simulink model "twolinkarm"  (R2017a)
settings: Solver=VariableStepAuto  StartTime=0.0  StopTime=tTotal  FixedStep=1e-6  MinStep=1e-8  RelTol=1e-3
values from neighbouring files (symbols this model uses):
  a1_val = 0.05    [twolinkarm_init.m]
  a2_val = 0.05    [twolinkarm_init.m]
  Jm = 3.2284E-6    (= 3.2284e-06)    [twolinkarm_init.m]
  lC1_val = a1_val/2    (= 0.025)    [twolinkarm_init.m]
  lC2_val = a2_val/2    (= 0.025)    [twolinkarm_init.m]
  mL1_val = 0.01    [twolinkarm_init.m]
  mL2_val = 0.01    [twolinkarm_init.m]
  ts = 0.1    [twolinkarm_init.m]
  V = 7.4    [twolinkarm_init.m]
  Y = simplify(Y)    [twolinkarm_DPI1.m]    (also in twolinkarm_DPI2.m = subs(Y, [lC1, lC2],[0.5*a1, 0.5*a2]); twolinkarm_init.m = subs(Y,      [a1, a2, lC1, lC2, k1, k2],      [a1_val, a2_va)
undefined symbols (not defined in the file or in its folder): Ry, X, Z
libraries: sm_lib x13, nesl_utility x11, fl_lib x10, elec_lib x2
settings Model: Creator=ashlin  LastModifiedBy=ashlin
settings SolverCC: ZeroCrossAlgorithm=Adaptive
settings DataIOCC: SaveFormat=Array
settings DiagnosticsConfigSet: SimMechanicsUnconnectedFramePorts=none  SimMechanicsUnconnectedGeometryPorts=none

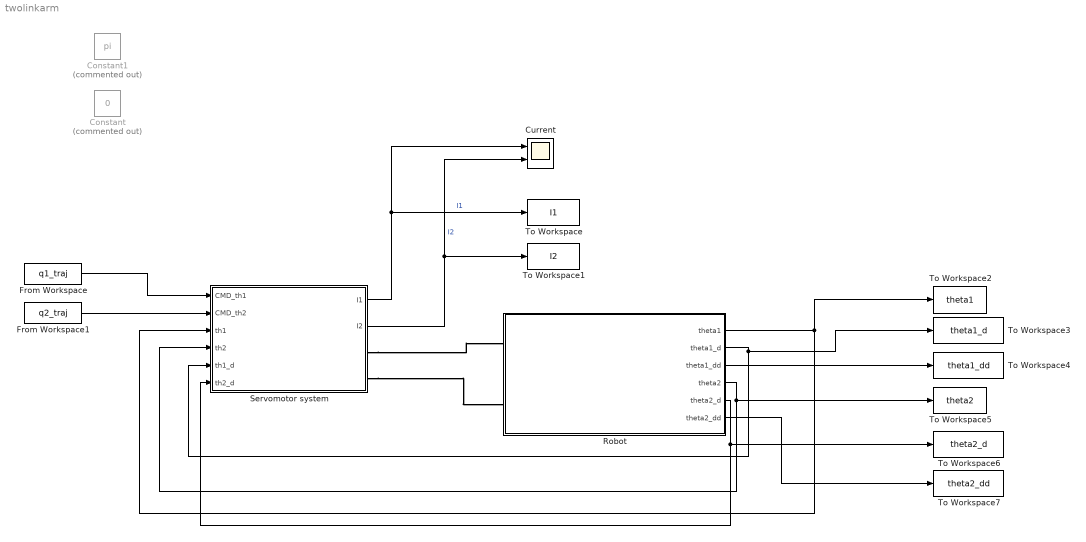
== system twolinkarm ==
  Constant : Constant  Commented=on  Value=0
  Constant1 : Constant  Commented=on  Value=pi
  Current : Scope  NumInputPorts=2
  From Workspace : FromWorkspace  VariableName=q1_traj  SampleTime=0
  From Workspace1 : FromWorkspace  VariableName=q2_traj  SampleTime=0
  Robot : Subsystem
  Servomotor system : Subsystem
  To Workspace : ToWorkspace  VariableName=I1  SaveFormat=Timeseries  SampleTime=ts
  To Workspace1 : ToWorkspace  VariableName=I2  SaveFormat=Timeseries  SampleTime=ts
  To Workspace2 : ToWorkspace  VariableName=theta1  SaveFormat=Timeseries  SampleTime=ts
  To Workspace3 : ToWorkspace  VariableName=theta1_d  SaveFormat=Timeseries  SampleTime=ts
  To Workspace4 : ToWorkspace  VariableName=theta1_dd  SaveFormat=Timeseries  SampleTime=ts
  To Workspace5 : ToWorkspace  VariableName=theta2  SaveFormat=Timeseries  SampleTime=ts
  To Workspace6 : ToWorkspace  VariableName=theta2_d  SaveFormat=Timeseries  SampleTime=ts
  To Workspace7 : ToWorkspace  VariableName=theta2_dd  SaveFormat=Timeseries  SampleTime=ts
  wires:
  Servomotor system/1(I1) -> To Workspace/1, Current/1  "I1"
  Servomotor system/2(I2) -> To Workspace1/1, Current/2  "I2"
  Robot/1(theta1) -> To Workspace2/1, Servomotor system/3(th1)
  Robot/2(theta1_d) -> To Workspace3/1, Servomotor system/5(th1_d)
  Robot/3(theta1_dd) -> To Workspace4/1
  Robot/5(theta2_d) -> To Workspace6/1, Servomotor system/6(th2_d)
  Robot/6(theta2_dd) -> To Workspace7/1
  Robot/4(theta2) -> Servomotor system/4(th2), To Workspace5/1
  From Workspace/1 -> Servomotor system/1(CMD_th1)
  From Workspace1/1 -> Servomotor system/2(CMD_th2)
  connections:
  Servomotor system/RConn1 -- Robot/LConn1
  Servomotor system/RConn2 -- Robot/LConn2

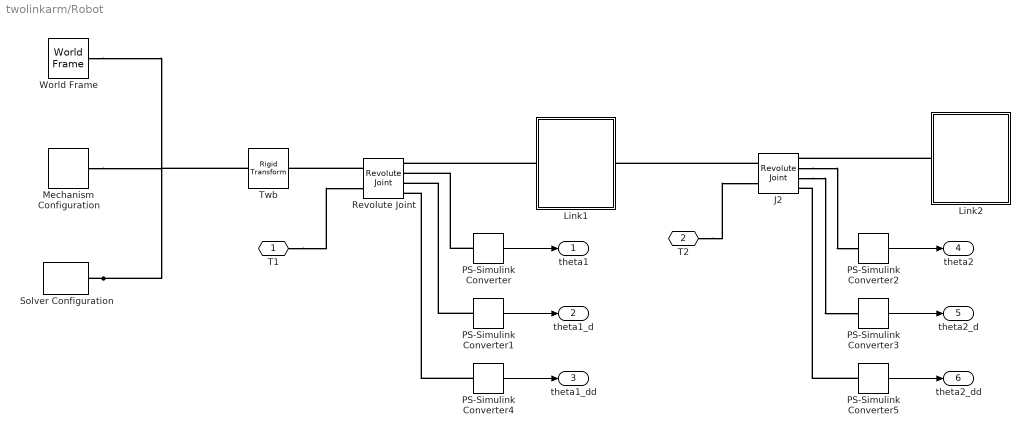
== system twolinkarm/Robot ==
  J2 : sm_lib/Joints/Revolute Joint  SenseConstraintForce=off  SenseConstraintForceX=off  SenseConstraintForceY=off  SenseConstraintForceZ=off  SenseConstraintTorque=off  SenseConstraintTorqueX=off  SenseConstraintTorqueY=off  SenseConstraintTorqueZ=off  SenseTotalForce=off  SenseTotalForceX=off  SenseTotalForceY=off  SenseTotalForceZ=off  SenseTotalTorque=off  SenseTotalTorqueX=off  SenseTotalTorqueY=off  SenseTotalTorqueZ=off  CompositeWrenchDir=FollowerOnBase  CompositeWrenchFrame=BaseFrame  EquilibriumPosition=0  EquilibriumPositionUnits=deg  SpringStiffness=0  SpringStiffnessUnits=N*m/deg  DampingCoefficient=0  DampingCoefficientUnits=N*m/(deg/s)  TorqueActuationMode=InputTorque  MotionActuationMode=ComputedMotion  SensePosition=on  SenseVelocity=on  SenseAcceleration=on  SenseTorqueForce=off  PositionTargetSpecify=off  PositionTargetPriority=High  PositionTargetValue=0  PositionTargetValueUnits=deg  VelocityTargetSpecify=off  VelocityTargetPriority=High  VelocityTargetValue=0  VelocityTargetValueUnits=deg/s
  Link1 : Subsystem
  Link2 : Subsystem
  Mechanism Configuration : sm_lib/Utilities/Mechanism Configuration  UniformGravity=Constant  GravityVector=[0 -9.81 0]  GravityUnits=m/s^2  LinearizationDelta=0.001
  PS-Simulink Converter{,1..5} (6 alike) : nesl_utility/PS-Simulink Converter  PhysicalDomain=network_engine_domain  SubClassName=ps_output  LeftPortType=input  RightPortType=output  PseudoPeriodic=off  Frequencies=[]  Unit=1  AffineConversion=off
  Revolute Joint : sm_lib/Joints/Revolute Joint  SenseConstraintForce=off  SenseConstraintForceX=off  SenseConstraintForceY=off  SenseConstraintForceZ=off  SenseConstraintTorque=off  SenseConstraintTorqueX=off  SenseConstraintTorqueY=off  SenseConstraintTorqueZ=off  SenseTotalForce=off  SenseTotalForceX=off  SenseTotalForceY=off  SenseTotalForceZ=off  SenseTotalTorque=off  SenseTotalTorqueX=off  SenseTotalTorqueY=off  SenseTotalTorqueZ=off  CompositeWrenchDir=FollowerOnBase  CompositeWrenchFrame=BaseFrame  EquilibriumPosition=0  EquilibriumPositionUnits=deg  SpringStiffness=0  SpringStiffnessUnits=N*m/deg  DampingCoefficient=0  DampingCoefficientUnits=N*m/(deg/s)  TorqueActuationMode=InputTorque  MotionActuationMode=ComputedMotion  SensePosition=on  SenseVelocity=on  SenseAcceleration=on  SenseTorqueForce=off  PositionTargetSpecify=off  PositionTargetPriority=High  PositionTargetValue=0  PositionTargetValueUnits=deg  VelocityTargetSpecify=off  VelocityTargetPriority=High  VelocityTargetValue=0  VelocityTargetValueUnits=deg/s
  Solver Configuration : nesl_utility/Solver Configuration  PhysicalDomain=network_engine_domain  SubClassName=solver  LeftPortType=input  RightPortType=generic  Accelerate=off  Tones=[]  Harmonics=[]  SimulateNoise=off  Profile=off  UseLocalSampling=off  EnableSwitchedLinearOptims=on  FrequencyDomain=off  UseCCode=off  RelTol=0.001  AbsTol=1e-06  MinStep=1e-09  ToWorkspace=off  RevertToSquareIcSolve=off  NumHomotopyIterations=100  PhasorMode=off  PhasorModeNumHarmonics=1  OverrideAbsTol=off  DoDC=off  ResidualTolerance=1e-04  UseLocalSolver=off  LocalSolverChoice=NE_BACKWARD_EULER_ADVANCER  LocalSolverSampleTime=0.001  DoFixedCost=off  MaxNonlinIter=3  MaxModeIter=2  LinearAlgebra=Sparse  DelaysMemoryBudget=1024  AutomaticFiltering=on  FilteringTimeConstant=0.001
  Twb : sm_lib/Frames and Transforms/Rigid Transform  TranslationMethod=None  TranslationStandardOffset=0  TranslationLengthUnit=m  TranslationStandardAxis=+Z  TranslationCartesianOffset=[0 0 0]  TranslationROffset=0  TranslationROffsetUnits=m  TranslationZOffset=0  TranslationZOffsetUnits=m  TranslationThetaOffset=0  TranslationThetaOffsetUnits=deg  RotationMethod=None  RotationAngleUnits=deg  RotationStandardAxis=+Z  RotationAngle=0.0  RotationArbitraryAxis=[0 0 1]  FollAlignAxisA=+X  BaseAlignAxisA=+Y  FollAlignAxisB=+Y  BaseAlignAxisB=+Z  RotationSequenceAxes=FollowerAxes  RotationSequence=XYX  RotationSequenceAngles=[0 0 0]  RotationSequenceAnglesUnits=deg  RotationMatrix=eye(3,3)
  World Frame : sm_lib/Frames and Transforms/World Frame
  T1 : PMIOPort  Port=1  Side=Left
  T2 : PMIOPort  Port=2  Side=Left
  theta1 : Outport
  theta1_d : Outport  Port=2
  theta1_dd : Outport  Port=3
  theta2 : Outport  Port=4
  theta2_d : Outport  Port=5
  theta2_dd : Outport  Port=6
  wires:
  PS-Simulink Converter/1 -> theta1/1
  PS-Simulink Converter1/1 -> theta1_d/1
  PS-Simulink Converter3/1 -> theta2_d/1
  PS-Simulink Converter2/1 -> theta2/1
  PS-Simulink Converter4/1 -> theta1_dd/1
  PS-Simulink Converter5/1 -> theta2_dd/1
  connections:
  Solver Configuration/RConn1 -- World Frame/RConn1 -- Twb/LConn1 -- Mechanism Configuration/RConn1
  PS-Simulink Converter/LConn1 -- Revolute Joint/RConn2
  T1/RConn1 -- Revolute Joint/LConn2
  Link1/LConn1 -- Revolute Joint/RConn1
  Revolute Joint/LConn1 -- Twb/RConn1
  J2/LConn1 -- Link1/RConn1
  T2/RConn1 -- J2/LConn2
  Link2/LConn1 -- J2/RConn1
  PS-Simulink Converter1/LConn1 -- Revolute Joint/RConn3
  J2/RConn2 -- PS-Simulink Converter2/LConn1
  J2/RConn3 -- PS-Simulink Converter3/LConn1
  PS-Simulink Converter4/LConn1 -- Revolute Joint/RConn4
  PS-Simulink Converter5/LConn1 -- J2/RConn4

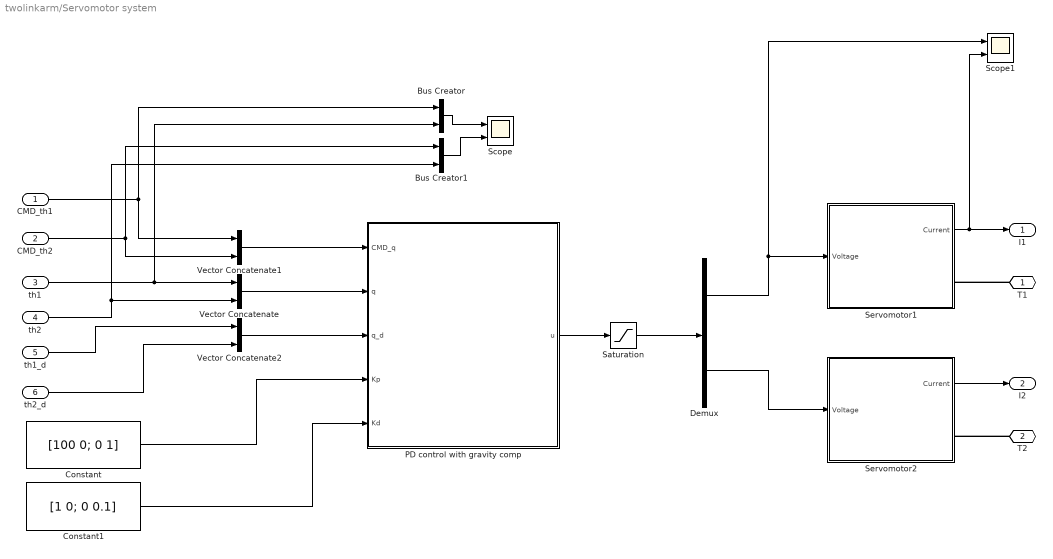
== system twolinkarm/Servomotor system ==
  CMD_th1 : Inport
  CMD_th2 : Inport  Port=2
  th1 : Inport  Port=3
  th2 : Inport  Port=4
  th1_d : Inport  Port=5
  th2_d : Inport  Port=6
  Bus Creator : BusCreator  Inputs=2
  Bus Creator1 : BusCreator  Inputs=2
  Constant : Constant  Value=[100 0; 0 1]
  Constant1 : Constant  Value=[1 0; 0 0.1]
  Demux : Demux  Outputs=2
  PD control with gravity comp : Subsystem
  Saturation : Saturate  UpperLimit=[V; V]  LowerLimit=[-V; -V]
  Scope : Scope  NumInputPorts=2
  Scope1 : Scope  NumInputPorts=2
  Servomotor1 : Subsystem
  Servomotor2 : Subsystem
  Vector Concatenate : Concatenate
  Vector Concatenate1 : Concatenate
  Vector Concatenate2 : Concatenate
  T1 : PMIOPort  Port=1  Side=Right
  T2 : PMIOPort  Port=2  Side=Right
  I1 : Outport
  I2 : Outport  Port=2
  wires:
  th1/1 -> Vector Concatenate/1, Bus Creator/2
  CMD_th1/1 -> Vector Concatenate1/1, Bus Creator/1
  Servomotor1/1(Current) -> Scope1/2, I1/1
  CMD_th2/1 -> Vector Concatenate1/2, Bus Creator1/1
  Servomotor2/1(Current) -> I2/1
  Demux/2 -> Servomotor2/1(Voltage)
  th2/1 -> Bus Creator1/2, Vector Concatenate/2
  Bus Creator1/1 -> Scope/2
  Bus Creator/1 -> Scope/1
  PD control with gravity comp/1(u) -> Saturation/1
  Vector Concatenate/1 -> PD control with gravity comp/2(q)
  Vector Concatenate1/1 -> PD control with gravity comp/1(CMD_q)
  Vector Concatenate2/1 -> PD control with gravity comp/3(q_d)
  th2_d/1 -> Vector Concatenate2/2
  th1_d/1 -> Vector Concatenate2/1
  Constant/1 -> PD control with gravity comp/4(Kp)
  Constant1/1 -> PD control with gravity comp/5(Kd)
  Demux/1 -> Scope1/1, Servomotor1/1(Voltage)
  Saturation/1 -> Demux/1
  connections:
  T1/RConn1 -- Servomotor1/RConn1
  T2/RConn1 -- Servomotor2/RConn1

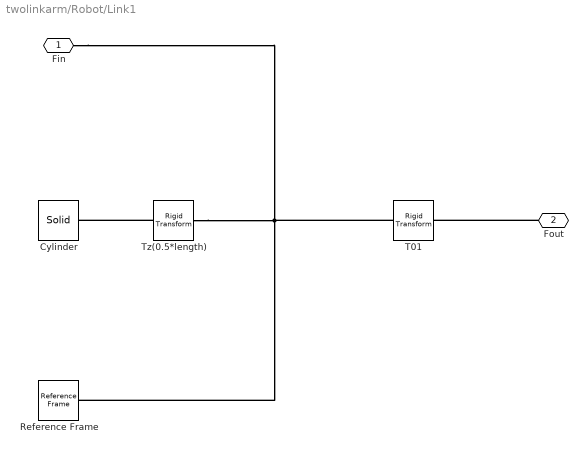
== system twolinkarm/Robot/Link1 ==
  Cylinder : sm_lib/Body Elements/Solid  InertiaType=CalculateFromGeometry  Mass=1  MassUnits=kg  CenterOfMass=[0 0 0]  CenterOfMassUnits=m  MomentsOfInertia=[1 1 1]  MomentsOfInertiaUnits=kg*m^2  ProductsOfInertia=[1 1 1]  ProductsOfInertiaUnits=kg*m^2  DensityBased=on  Density=density  DensityUnits=kg/m^3  DoExposeReferenceFrame=on  SerializedFrames=<Frames/>  GraphicType=FromGeometry  MarkerShape=Sphere  MarkerSize=10  GraphicVisPropType=SimpleVisualProperties  GraphicDiffuseColor=[0.0 1.0 0.4]  GraphicSpecularColor=[0.5 0.5 0.5 1.0]  GraphicAmbientColor=[0.15 0.15 0.15 1.0]  GraphicEmissiveColor=[0.0 0.0 0.0 1.0]  GraphicShininess=75  GraphicOpacity=1.0  GeometryShape=Cylinder  RectangleSize=[1 1]  RectangleSizeUnits=m  BrickDimensions=[1 1 1]  BrickDimensionUnits=m  CylinderRadius=rLink  CylinderRadiusUnits=m  CylinderLength=a1_val  CylinderLengthUnits=m  SphereRadius=1  SphereRadiusUnits=m  EllipsoidRadii=[1 1 1]  EllipsoidRadiiUnits=m  ExtrusionCrossSection=[1 1; -1 1; -1 -1; 1 -1]  ExtrusionCrossSectionUnits=m  ExtrusionLength=1  ExtrusionLengthUnits=m  PolygonNumSides=3  PolygonOuterRadius=1  PolygonOuterRadiusUnits=m  ExtGeomFileType=STEP  ExtGeomFileUnits=m  RevolutionCrossSection=[1 1; 1 -1; 2 -1; 2 1]  RevolutionCrossSectionUnits=m  RevolutionExtent=Full  RevolutionAngle=180  RevolutionAngleUnits=deg
  Reference Frame : sm_lib/Frames and Transforms/Reference Frame
  T01 : sm_lib/Frames and Transforms/Rigid Transform  TranslationMethod=Cartesian  TranslationStandardOffset=0.1/2  TranslationLengthUnit=m  TranslationStandardAxis=+Z  TranslationCartesianOffset=[a1_val 0 0]  TranslationROffset=0  TranslationROffsetUnits=m  TranslationZOffset=0  TranslationZOffsetUnits=m  TranslationThetaOffset=0  TranslationThetaOffsetUnits=deg  RotationMethod=RotationMatrix  RotationAngleUnits=deg  RotationStandardAxis=+Y  RotationAngle=90  RotationArbitraryAxis=[0 0 1]  FollAlignAxisA=+X  BaseAlignAxisA=+Y  FollAlignAxisB=+Y  BaseAlignAxisB=+Z  RotationSequenceAxes=FollowerAxes  RotationSequence=XYX  RotationSequenceAngles=[0 0 0]  RotationSequenceAnglesUnits=deg  RotationMatrix=eye(3,3)
  Tz(0.5*length) : sm_lib/Frames and Transforms/Rigid Transform  TranslationMethod=Cartesian  TranslationStandardOffset=0  TranslationLengthUnit=m  TranslationStandardAxis=-X  TranslationCartesianOffset=[ 0 0 -a1_val/2]  TranslationROffset=0  TranslationROffsetUnits=m  TranslationZOffset=0  TranslationZOffsetUnits=m  TranslationThetaOffset=0  TranslationThetaOffsetUnits=deg  RotationMethod=RotationMatrix  RotationAngleUnits=deg  RotationStandardAxis=+Z  RotationAngle=0.0  RotationArbitraryAxis=[0 0 1]  FollAlignAxisA=+X  BaseAlignAxisA=+Y  FollAlignAxisB=+Y  BaseAlignAxisB=+Z  RotationSequenceAxes=FollowerAxes  RotationSequence=XYX  RotationSequenceAngles=[0 0 0]  RotationSequenceAnglesUnits=deg  RotationMatrix=Ry(pi/2)
  Fin : PMIOPort  Port=1  Side=Left
  Fout : PMIOPort  Port=2  Side=Right
  connections:
  Tz(0.5*length)/LConn1 -- Cylinder/RConn1
  Fin/RConn1 -- T01/LConn1 -- Tz(0.5*length)/RConn1 -- Reference Frame/RConn1
  Fout/RConn1 -- T01/RConn1

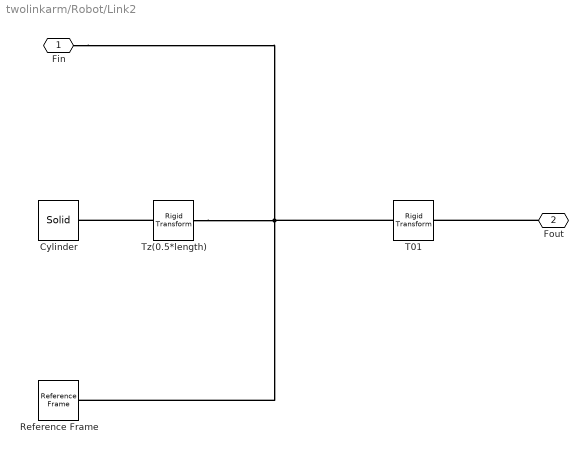
== system twolinkarm/Robot/Link2 ==
  Cylinder : sm_lib/Body Elements/Solid  InertiaType=CalculateFromGeometry  Mass=1  MassUnits=kg  CenterOfMass=[0 0 0]  CenterOfMassUnits=m  MomentsOfInertia=[1 1 1]  MomentsOfInertiaUnits=kg*m^2  ProductsOfInertia=[1 1 1]  ProductsOfInertiaUnits=kg*m^2  DensityBased=on  Density=density  DensityUnits=kg/m^3  DoExposeReferenceFrame=on  SerializedFrames=<Frames/>  GraphicType=FromGeometry  MarkerShape=Sphere  MarkerSize=10  GraphicVisPropType=SimpleVisualProperties  GraphicDiffuseColor=[0.0 1.0 0.4]  GraphicSpecularColor=[0.5 0.5 0.5 1.0]  GraphicAmbientColor=[0.15 0.15 0.15 1.0]  GraphicEmissiveColor=[0.0 0.0 0.0 1.0]  GraphicShininess=75  GraphicOpacity=1.0  GeometryShape=Cylinder  RectangleSize=[1 1]  RectangleSizeUnits=m  BrickDimensions=[1 1 1]  BrickDimensionUnits=m  CylinderRadius=rLink  CylinderRadiusUnits=m  CylinderLength=a2_val  CylinderLengthUnits=m  SphereRadius=1  SphereRadiusUnits=m  EllipsoidRadii=[1 1 1]  EllipsoidRadiiUnits=m  ExtrusionCrossSection=[1 1; -1 1; -1 -1; 1 -1]  ExtrusionCrossSectionUnits=m  ExtrusionLength=1  ExtrusionLengthUnits=m  PolygonNumSides=3  PolygonOuterRadius=1  PolygonOuterRadiusUnits=m  ExtGeomFileType=STEP  ExtGeomFileUnits=m  RevolutionCrossSection=[1 1; 1 -1; 2 -1; 2 1]  RevolutionCrossSectionUnits=m  RevolutionExtent=Full  RevolutionAngle=180  RevolutionAngleUnits=deg
  Reference Frame : sm_lib/Frames and Transforms/Reference Frame
  T01 : sm_lib/Frames and Transforms/Rigid Transform  TranslationMethod=Cartesian  TranslationStandardOffset=0.1/2  TranslationLengthUnit=m  TranslationStandardAxis=+Z  TranslationCartesianOffset=[a2_val 0 0]  TranslationROffset=0  TranslationROffsetUnits=m  TranslationZOffset=0  TranslationZOffsetUnits=m  TranslationThetaOffset=0  TranslationThetaOffsetUnits=deg  RotationMethod=RotationMatrix  RotationAngleUnits=deg  RotationStandardAxis=+Y  RotationAngle=90  RotationArbitraryAxis=[0 0 1]  FollAlignAxisA=+X  BaseAlignAxisA=+Y  FollAlignAxisB=+Y  BaseAlignAxisB=+Z  RotationSequenceAxes=FollowerAxes  RotationSequence=XYX  RotationSequenceAngles=[0 0 0]  RotationSequenceAnglesUnits=deg  RotationMatrix=eye(3,3)
  Tz(0.5*length) : sm_lib/Frames and Transforms/Rigid Transform  TranslationMethod=StandardAxis  TranslationStandardOffset=a2_val/2  TranslationLengthUnit=m  TranslationStandardAxis=-Z  TranslationCartesianOffset=[ 0 0 -0.25]  TranslationROffset=0  TranslationROffsetUnits=m  TranslationZOffset=0  TranslationZOffsetUnits=m  TranslationThetaOffset=0  TranslationThetaOffsetUnits=deg  RotationMethod=RotationMatrix  RotationAngleUnits=deg  RotationStandardAxis=+Z  RotationAngle=0.0  RotationArbitraryAxis=[0 0 1]  FollAlignAxisA=+X  BaseAlignAxisA=+Y  FollAlignAxisB=+Y  BaseAlignAxisB=+Z  RotationSequenceAxes=FollowerAxes  RotationSequence=XYX  RotationSequenceAngles=[0 0 0]  RotationSequenceAnglesUnits=deg  RotationMatrix=Ry(pi/2)
  Fin : PMIOPort  Port=1  Side=Left
  Fout : PMIOPort  Port=2  Side=Right
  connections:
  Tz(0.5*length)/LConn1 -- Cylinder/RConn1
  Fin/RConn1 -- T01/LConn1 -- Tz(0.5*length)/RConn1 -- Reference Frame/RConn1
  Fout/RConn1 -- T01/RConn1

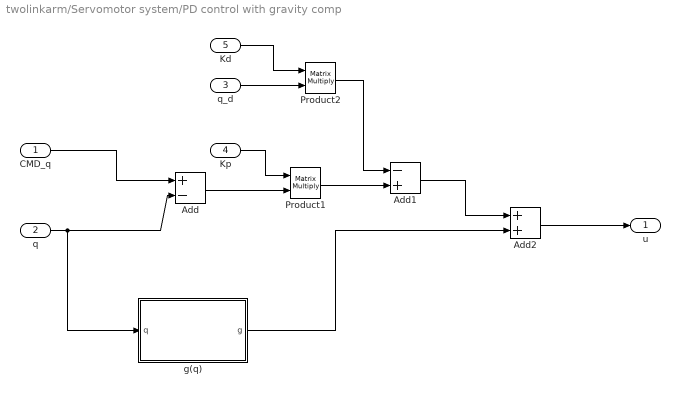
== system twolinkarm/Servomotor system/PD control with gravity comp ==
  CMD_q : Inport  PortDimensions=[2 1]
  q : Inport  Port=2  PortDimensions=[2 1]
  q_d : Inport  Port=3  PortDimensions=[2 1]
  Kp : Inport  Port=4  PortDimensions=[2 2]
  Kd : Inport  Port=5  PortDimensions=[2 2]
  Add : Sum  Inputs=+-
  Add1 : Sum  Inputs=-+
  Add2 : Sum
  Product1 : Product  Multiplication=Matrix(*)
  Product2 : Product  Multiplication=Matrix(*)
  g(q) : Subsystem
  u : Outport
  wires:
  q/1 -> g(q)/1(q), Add/2
  CMD_q/1 -> Add/1
  Add/1 -> Product1/2
  Kp/1 -> Product1/1
  Product1/1 -> Add1/2
  Add1/1 -> Add2/1
  Add2/1 -> u/1
  Product2/1 -> Add1/1
  g(q)/1(g) -> Add2/2
  Kd/1 -> Product2/1
  q_d/1 -> Product2/2

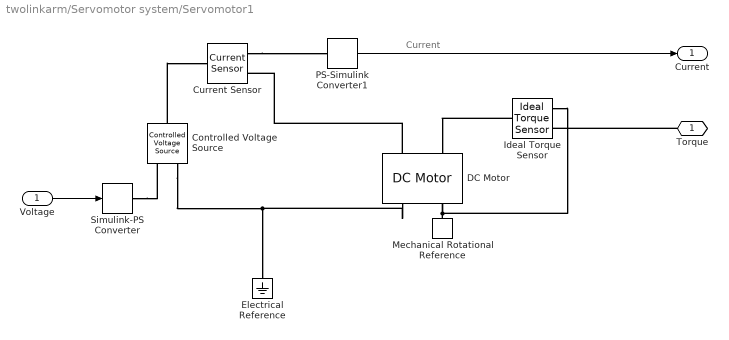
== system twolinkarm/Servomotor system/Servomotor1 ==
  note: Current
  Voltage : Inport
  Controlled Voltage Source : fl_lib/Electrical/Electrical Sources/Controlled Voltage Source
  Current Sensor : fl_lib/Electrical/Electrical Sensors/Current Sensor
  DC Motor : elec_lib/Actuators & Drivers/Rotational Actuators/DC Motor  parameterization=2  Ra=Ra Ohm  La=La H  emf_or_torque=1  Kv=Kemf V/rpm  Ki=6.876e-4 N*m/A  T_stall=Tstall N*m  w_max=Wnoload rpm  w_rated=1.5e+4 rpm  P_rated=0.08 W  V_rated=V V  J=Jm g*cm^2  lam_param=1  lam=bm N*m/(rad/s)  i_noload=0 A  V_i_noload=1.5 V  speed0=0 rpm  alpha=0.00393 1/K  Tmeas=25 degC  thermal_mass=100 J/K  initial_temperature=25 degC
  Electrical Reference : fl_lib/Electrical/Electrical Elements/Electrical Reference
  Ideal Torque Sensor : fl_lib/Mechanical/Mechanical Sensors/Ideal Torque Sensor
  Mechanical Rotational Reference : fl_lib/Mechanical/Rotational Elements/Mechanical Rotational Reference
  PS-Simulink Converter1 : nesl_utility/PS-Simulink Converter  PhysicalDomain=network_engine_domain  SubClassName=ps_output  LeftPortType=input  RightPortType=output  PseudoPeriodic=off  Frequencies=[]  Unit=1  AffineConversion=off
  Simulink-PS Converter : nesl_utility/Simulink-PS Converter  PhysicalDomain=network_engine_domain  SubClassName=ps_input  LeftPortType=input  RightPortType=output  PseudoPeriodic=off  Frequencies=[]  NoiseDistribution=none  NoiseParameters=[]  Unit=1  AffineConversion=off  FilteringAndDerivatives=provide  SimscapeFilterOrder=1  InputFilterTimeConstant=0.001  UdotUserProvided=0
  Torque : PMIOPort  Port=1  Side=Right
  Current : Outport
  wires:
  Voltage/1 -> Simulink-PS Converter/1
  PS-Simulink Converter1/1 -> Current/1
  connections:
  Controlled Voltage Source/RConn2 -- DC Motor/RConn1 -- Electrical Reference/LConn1
  Current Sensor/RConn1 -- PS-Simulink Converter1/LConn1
  Controlled Voltage Source/LConn1 -- Current Sensor/LConn1
  DC Motor/LConn1 -- Current Sensor/RConn2
  Simulink-PS Converter/RConn1 -- Controlled Voltage Source/RConn1
  Mechanical Rotational Reference/LConn1 -- Ideal Torque Sensor/RConn1 -- DC Motor/RConn2
  Ideal Torque Sensor/LConn1 -- DC Motor/LConn2
  Torque/RConn1 -- Ideal Torque Sensor/RConn2

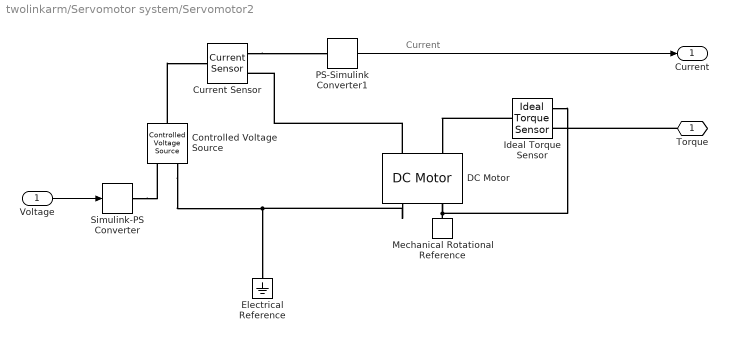
== system twolinkarm/Servomotor system/Servomotor2 ==
  note: Current
  Voltage : Inport
  Controlled Voltage Source : fl_lib/Electrical/Electrical Sources/Controlled Voltage Source
  Current Sensor : fl_lib/Electrical/Electrical Sensors/Current Sensor
  DC Motor : elec_lib/Actuators & Drivers/Rotational Actuators/DC Motor  parameterization=2  Ra=Ra Ohm  La=La H  emf_or_torque=1  Kv=Kemf V/rpm  Ki=6.876e-4 N*m/A  T_stall=4.903325 N*m  w_max=58.82 rpm  w_rated=1.5e+4 rpm  P_rated=0.08 W  V_rated=7.4 V  J=Jm g*cm^2  lam_param=1  lam=bm N*m/(rad/s)  i_noload=0 A  V_i_noload=1.5 V  speed0=0 rpm  alpha=0.00393 1/K  Tmeas=25 degC  thermal_mass=100 J/K  initial_temperature=25 degC
  Electrical Reference : fl_lib/Electrical/Electrical Elements/Electrical Reference
  Ideal Torque Sensor : fl_lib/Mechanical/Mechanical Sensors/Ideal Torque Sensor
  Mechanical Rotational Reference : fl_lib/Mechanical/Rotational Elements/Mechanical Rotational Reference
  PS-Simulink Converter1 : nesl_utility/PS-Simulink Converter  PhysicalDomain=network_engine_domain  SubClassName=ps_output  LeftPortType=input  RightPortType=output  PseudoPeriodic=off  Frequencies=[]  Unit=1  AffineConversion=off
  Simulink-PS Converter : nesl_utility/Simulink-PS Converter  PhysicalDomain=network_engine_domain  SubClassName=ps_input  LeftPortType=input  RightPortType=output  PseudoPeriodic=off  Frequencies=[]  NoiseDistribution=none  NoiseParameters=[]  Unit=1  AffineConversion=off  FilteringAndDerivatives=provide  SimscapeFilterOrder=1  InputFilterTimeConstant=0.001  UdotUserProvided=0
  Torque : PMIOPort  Port=1  Side=Right
  Current : Outport
  wires:
  Voltage/1 -> Simulink-PS Converter/1
  PS-Simulink Converter1/1 -> Current/1
  connections:
  Controlled Voltage Source/RConn2 -- DC Motor/RConn1 -- Electrical Reference/LConn1
  Current Sensor/RConn1 -- PS-Simulink Converter1/LConn1
  Controlled Voltage Source/LConn1 -- Current Sensor/LConn1
  DC Motor/LConn1 -- Current Sensor/RConn2
  Simulink-PS Converter/RConn1 -- Controlled Voltage Source/RConn1
  Mechanical Rotational Reference/LConn1 -- Ideal Torque Sensor/RConn1 -- DC Motor/RConn2
  Ideal Torque Sensor/LConn1 -- DC Motor/LConn2
  Torque/RConn1 -- Ideal Torque Sensor/RConn2

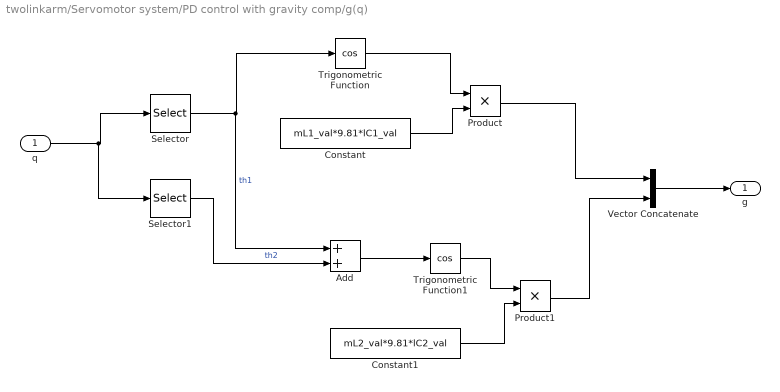
== system twolinkarm/Servomotor system/PD control with gravity comp/g(q) ==
  q : Inport
  Add : Sum
  Constant : Constant  Value=mL1_val*9.81*lC1_val
  Constant1 : Constant  Value=mL2_val*9.81*lC2_val
  Product : Product
  Product1 : Product
  Selector : Selector  InputPortWidth=2  IndexOptions=Index vector (dialog)  Indices=1  OutputSizes=1
  Selector1 : Selector  InputPortWidth=2  IndexOptions=Index vector (dialog)  Indices=2  OutputSizes=1
  Trigonometric Function : Trigonometry  Operator=cos
  Trigonometric Function1 : Trigonometry  Operator=cos
  Vector Concatenate : Concatenate
  g : Outport  PortDimensions=[ 2 1]
  wires:
  Trigonometric Function/1 -> Product/1
  Constant/1 -> Product/2
  q/1 -> Selector1/1, Selector/1
  Selector/1 -> Add/1, Trigonometric Function/1  "th1"
  Selector1/1 -> Add/2  "th2"
  Add/1 -> Trigonometric Function1/1
  Trigonometric Function1/1 -> Product1/1
  Constant1/1 -> Product1/2
  Product/1 -> Vector Concatenate/1
  Product1/1 -> Vector Concatenate/2
  Vector Concatenate/1 -> g/1
